simulink library "NxtrNvM"  (R2013b)
settings: Solver=ode45  StartTime=0.0  StopTime=10.0  RelTol=1e-3
settings Model: Creator=cz7lt6  LastModifiedBy=DZ1YRM

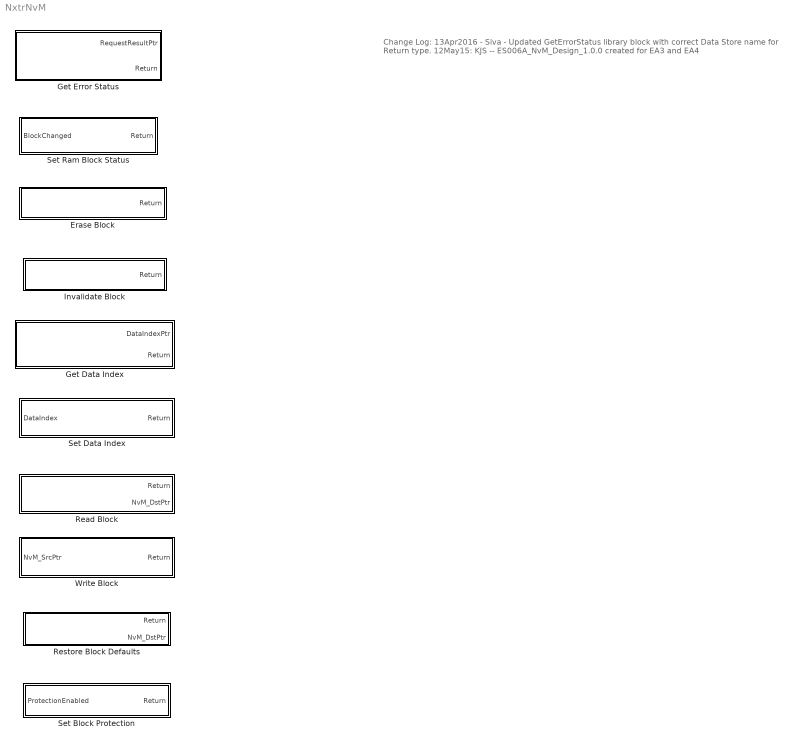
== system NxtrNvM ==
  note: Change Log:
      |
      |  13Apr2016 - Siva - Updated GetErrorStatus library block with correct Data Store name for Return type.
      |
      | 12May15: KJS -- ES006A_NvM_Design_1.0.0 created for EA3 and EA4
  Erase Block : Subsystem  mask(NvM EraseBlock){FuncName=Erase Block, NvMBlockName=, VoidFuncRtn=off, Return_DSN=NvMEraseBlk_Return}
      mask prompts: FuncName "%<FuncName>"; NvMBlockName "NvM Block Name"; VoidFuncRtn "Cast Function Return to Void"; Return_DSN "Data Store for Return"
      mask help: Click on Help for more details with respect to this function.
      mask init:
      | blk = [gcb '/Return'];
      | blkPos = get_param(blk, 'Position');
      | blkOri = get_param(blk, 'Orientation');
      | blkType = get_param(blk, 'BlockType');
      | 
      | if VoidFuncRtn
      |     if strcmp(blkType,'Outport')
      |         % Remove port and replace with terminator in the same location
      |         delete_block(blk);
      |         add_block('built-in/Terminator',blk,'Position',blkPos,...
      |                   'Orientation',blkOri);
      |         % Remove port and replace with terminator in the same location
      |         add_block('built-in/DataStoreMemory',[gcb '/Memory']);
      |         StoreName = get_param([gcb '/NvMEraseBlock_Return'],'DataStoreName');
      |         set_param([gcb '/Memory'],'DataStoreName',StoreName);
      |         
      |         % Add input port and terminate it
      |         add_block('built-in/Inport', [gcb '/CallFunction']);
      |         add_block('built-in/Terminator', [gcb '/CallFuncTerm']);
      |         add_line(gcb, 'CallFunction/1', 'CallFuncTerm/1',...
      |                  'autorouting', 'on');
      |         
      |         % Diable changes to Return data store
      |         set_param(gcb,'MaskEnableString','on,on,on,off');
      |     end
      | else
      |     if strcmp(blkType, 'Terminator')
      |         % Remove terminator and replace with outport
      |         delete_block(blk);
      |         add_block('built-in/Outport',blk,'Position',blkPos,...
      |                   'Orientation',blkOri);
      |         delete_block([gcb '/Memory']);
      |         
      |         %Remove input ports and connection
      |         delete_line(gcb, 'CallFunction/1', 'CallFuncTerm/1');
      |         delete_block([gcb '/CallFunction']);
      |         delete_block([gcb '/CallFuncTerm']);
      |         
      |         % Enable all fields in mask
      |         set_param(gcb,'MaskEnableString','on,on,on,on');
      |     end
      | end
      | %END%
      settings: AttributesFormatString=%<FuncName>
      mask Help: eval('web(NvMLibHelp(''EraseBlock.html''))')
      mask TypeOptions Return_DSN: NvMEraseBlock_Return/DataStoreName
      mask Display:
      | % Adjust ports based on mask configuration.
      | if VoidFuncRtn
      |     % No 'Return' port
      |     port_label('input',1,'CallFunction');
      | else
      |     port_label('output',1,'Return');
      | end
      | 
      | % Check NvM Block Name parameter
      | if isempty(NvMBlockName)
      |     NvMBlockName = 'Undefined NvM Block';
      |     color('red');
      | end
      | text(0.02,0.95,[NvMBlockName],...
      |      'horizontalAlignment', 'left',...
      |      'verticalAlignment','top');
  Get Data Index : Subsystem  mask(NvM GetDataIndex){FuncName=Get Data Index, NvMBlockName=, VoidFuncRtn=off, DataIndexPtr_DSN=DataIndexPtr, Return_DSN=NvMGDI_Return}
      mask prompts: FuncName "%<FuncName>"; NvMBlockName "NvM Block Name"; VoidFuncRtn "Cast Function Return to Void"; DataIndexPtr_DSN "Data Store for DataIndexPtr"; Return_DSN "Data Store for Return"
      mask help: Click on Help for more details with respect to this function.
      mask init:
      | blk = [gcb '/Return'];
      | blkPos = get_param(blk, 'Position');
      | blkOri = get_param(blk, 'Orientation');
      | blkType = get_param(blk, 'BlockType');
      | 
      | if VoidFuncRtn
      |     if strcmp(blkType,'Outport')
      |         % Remove port and replace with terminator in the same location
      |         delete_block(blk);
      |         add_block('built-in/Terminator',blk,'Position',blkPos,...
      |                   'Orientation',blkOri);
      |         
      |         % Add internal data store to prevent simulation errors
      |         add_block('built-in/DataStoreMemory',[gcb '/Memory']);
      |         
      |         % Give it the same name as the configured value
      |         StoreName = get_param([gcb '/NvMGDI_Return'],'DataStoreName');
      |         set_param([gcb '/Memory'],'DataStoreName',StoreName);
      | 
      |         % Turn off field in mask to prevent changes.
      |         set_param(gcb,'MaskEnableString','on,on,on,on,off')
      |     end
      | else
      |     if strcmp(blkType, 'Terminator')
      |         % Remove terminator and replace with outport
      |         delete_block(blk);
      |         add_block('built-in/Outport',blk,'Position',blkPos,...
      |                   'Orientation',blkOri);
      |         
      |         % Remove internal data store
      |         delete_block([gcb '/Memory']);
      |         
      |         % Enable field in mask to allow changes 
      |         set_param(gcb,'MaskEnableString','on,on,on,on,on')
      |     end
      | end
      settings: AttributesFormatString=%<FuncName>
      mask Help: eval('web(NvMLibHelp(''GetDataIndex.html''))')
      mask TypeOptions DataIndexPtr_DSN: NvMGDI_DataIndexPtr/DataStoreName
      mask TypeOptions Return_DSN: NvMGDI_Return/DataStoreName
      mask Display:
      | % Adjust ports based on mask configuration.
      | if VoidFuncRtn
      |     port_label('output',1,'DataIndexPtr');
      | else
      |     port_label('output',1,'DataIndexPtr');
      |     port_label('output',2,'Return');
      | end
      | 
      | % Check NvM Block Name parameter
      | if isempty(NvMBlockName)
      |     NvMBlockName = 'Undefined NvM Block';
      |     color('red');
      | end
      | text(0.02,0.95,[NvMBlockName],...
      |      'horizontalAlignment', 'left',...
      |      'verticalAlignment','top');
  Get Error Status : Subsystem  TreatAsAtomicUnit=on  mask(NvM GetErrorStatus){FuncName=Get Error Status, NvMBlockName=, VoidFuncRtn=off, ReqResPtr_DSN=NvMGES_ReqResPtr, Return_DSN=NvMGES_Return}
      mask prompts: FuncName "%<FuncName>"; NvMBlockName "NvM Block Name"; VoidFuncRtn "Cast Function Return to Void"; ReqResPtr_DSN "Data Store for ReqResPtr"; Return_DSN "Data Store for Return"
      mask help: Click on Help for more details with respect to this function.
      mask init:
      | blk = [gcb '/Return'];
      | blkPos = get_param(blk, 'Position');
      | blkOri = get_param(blk, 'Orientation');
      | blkType = get_param(blk, 'BlockType');
      | 
      | if VoidFuncRtn
      |     if strcmp(blkType,'Outport')
      |         % Remove port and replace with terminator in the same location
      |         delete_block(blk);
      |         add_block('built-in/Terminator',blk,'Position',blkPos,...
      |                   'Orientation',blkOri);
      |         % Add internal data store to prevent simulation errors
      |         add_block('built-in/DataStoreMemory',[gcb '/Memory']);
      |         
      |         % Give it the same name as the configured value
      |         StoreName = get_param([gcb '/NvMGES_Return'],'DataStoreName');
      |         set_param([gcb '/Memory'],'DataStoreName',StoreName);
      |         
      |         % Turn off field in mask to prevent changes.
      |         set_param(gcb,'MaskEnableString','on,on,on,on,off')
      |     end
      | else
      |     if strcmp(blkType, 'Terminator')
      |         % Remove terminator and replace with outport
      |         delete_block(blk);
      |         add_block('built-in/Outport',blk,'Position',blkPos,...
      |                   'Orientation',blkOri);
      |         
      |         % Remove internal data store
      |         delete_block([gcb '/Memory']);
      |         
      |         % Enable field in mask to allow changes 
      |         set_param(gcb,'MaskEnableString','on,on,on,on,on')
      |     end
      | end
      | %END%
      settings: AttributesFormatString=%<FuncName>
      mask Help: eval('web(NvMLibHelp(''GetErrorStatus.html''))')
      mask TypeOptions ReqResPtr_DSN: NvMGES_ReqResPtr/DataStoreName
      mask TypeOptions Return_DSN: NvMGES_Return/DataStoreName
      mask Display:
      | % Adjust ports based on mask configuration.
      | if VoidFuncRtn
      |     % No 'Return' port
      |     port_label('output',1,'ReqResPtr');
      | else
      |     port_label('output',1,'ReqResPtr');
      |     port_label('output',2,'Return');
      | end
      | 
      | % Check NvM Block Name parameter
      | if isempty(NvMBlockName)
      |     NvMBlockName = 'Undefined NvM Block';
      |     color('red');
      | end
      | text(0.02,0.95,[NvMBlockName],...
      |      'horizontalAlignment', 'left',...
      |      'verticalAlignment','top');
  Invalidate Block : Subsystem  mask(NvM InvalidateBlock){FuncName=Invalidate Block, NvMBlockName=, VoidFuncRtn=off, Return_DSN=NvMInvalidateBlk_Return}
      mask prompts: FuncName "%<FuncName>"; NvMBlockName "NvM Block Name"; VoidFuncRtn "Cast Function Return to Void"; Return_DSN "Data Store for Return"
      mask help: Click on Help for more details with respect to this function.
      mask init:
      | blk = [gcb '/Return'];
      | blkPos = get_param(blk, 'Position');
      | blkOri = get_param(blk, 'Orientation');
      | blkType = get_param(blk, 'BlockType');
      | 
      | if VoidFuncRtn
      |     if strcmp(blkType,'Outport')
      |         % Remove port and replace with terminator in the same location
      |         delete_block(blk);
      |         add_block('built-in/Terminator',blk,'Position',blkPos,...
      |                   'Orientation',blkOri);
      |         % Remove port and replace with terminator in the same location
      |         add_block('built-in/DataStoreMemory',[gcb '/Memory']);
      |         StoreName = get_param([gcb '/NvMInvalidateBlock_Return'],'DataStoreName');
      |         set_param([gcb '/Memory'],'DataStoreName',StoreName);
      |         
      |         % Add input port and terminate it
      |         add_block('built-in/Inport', [gcb '/CallFunction']);
      |         add_block('built-in/Terminator', [gcb '/CallFuncTerm']);
      |         add_line(gcb, 'CallFunction/1', 'CallFuncTerm/1',...
      |                  'autorouting', 'on');
      |         
      |         % Diable changes to Return data store
      |         set_param(gcb,'MaskEnableString','on,on,on,off');
      |     end
      | else
      |     if strcmp(blkType, 'Terminator')
      |         % Remove terminator and replace with outport
      |         delete_block(blk);
      |         add_block('built-in/Outport',blk,'Position',blkPos,...
      |                   'Orientation',blkOri);
      |         delete_block([gcb '/Memory']);
      |         
      |         %Remove input ports and connection
      |         delete_line(gcb, 'CallFunction/1', 'CallFuncTerm/1');
      |         delete_block([gcb '/CallFunction']);
      |         delete_block([gcb '/CallFuncTerm']);
      |         
      |         % Enable all fields in mask
      |         set_param(gcb,'MaskEnableString','on,on,on,on');
      |     end
      | end
      | %END%
      settings: AttributesFormatString=%<FuncName>
      mask Help: eval('web(NvMLibHelp(''InvalidateBlock.html''))')
      mask TypeOptions Return_DSN: NvMInvalidateBlock_Return/DataStoreName
      mask Display:
      | % Adjust ports based on mask configuration.
      | if VoidFuncRtn
      |     % No 'Return' port
      |     port_label('input',1,'CallFunction');
      | else
      |     port_label('output',1,'Return');
      | end
      | 
      | % Check NvM Block Name parameter
      | if isempty(NvMBlockName)
      |     NvMBlockName = 'Undefined NvM Block';
      |     color('red');
      | end
      | text(0.02,0.95,[NvMBlockName],...
      |      'horizontalAlignment', 'left',...
      |      'verticalAlignment','top');
  Read Block : Subsystem  mask(NvM ReadBlock){FuncName=Read Block, NvMBlockName=, VoidFuncRtn=off, NvMDstPtr_DSN=NvM_DstPtr, Return_DSN=NvMReadBlock_Return, NullPtr=off}
      mask prompts: FuncName "%<FuncName>"; NvMBlockName "NvM Block Name"; VoidFuncRtn "Cast Function Return to Void"; NvMDstPtr_DSN "Data Store for NvM_DstPtr"; Return_DSN "Data Store for Return"; NullPtr "Set Output to NULL_PTR"
      mask help: Click on Help for more details with respect to this function.
      mask init:
      | blk = [gcb '/Return'];
      | blkPos = get_param(blk, 'Position');
      | blkOri = get_param(blk, 'Orientation');
      | blkType = get_param(blk, 'BlockType');
      | 
      | if VoidFuncRtn
      |     if strcmp(blkType,'Outport')
      |         % Remove port and replace with terminator in the same location
      |         delete_block(blk);
      |         add_block('built-in/Terminator',blk,'Position',blkPos,...
      |                   'Orientation',blkOri);
      |               
      |         % Add internal data store to prevent simulation errors
      |         add_block('built-in/DataStoreMemory',[gcb '/Memory']);
      |         
      |         % Give it the same name as the configured value
      |         StoreName = get_param([gcb '/NvMReadBlock_Return'],'DataStoreName');
      |         set_param([gcb '/Memory'],'DataStoreName',StoreName);
      |         
      |         % Turn off field in mask to prevent changes.
      |         set_param(gcb,'MaskEnableString','on,on,on,on,off,on')
      |     end
      | else
      |     if strcmp(blkType, 'Terminator')
      |         % Remove terminator and replace with outport
      |         delete_block(blk);
      |         add_block('built-in/Outport',blk,'Position',blkPos,...
      |                   'Orientation',blkOri);
      |         
      |         % Remove internal data store
      |         delete_block([gcb '/Memory']);
      |         
      |         % Enable field in mask to allow changes 
      |         set_param(gcb,'MaskEnableString','on,on,on,on,on,on')
      |     end
      | end
      | 
      | blk = [gcb '/NvM_DstPtr'];
      | blkPos = get_param(blk, 'Position');
      | blkOri = get_param(blk, 'Orientation');
      | blkType = get_param(blk, 'BlockType');
      | 
      | if NullPtr
      |     if strcmp(blkType,'Outport')
      |         % Remove port and replace with terminator in the same location
      |         delete_block(blk);
      |         add_block('built-in/Terminator',blk,'Position',blkPos,...
      |                   'Orientation',blkOri);
      |               
      |         % Add internal data store to prevent simulation errors
      |         add_block('built-in/DataStoreMemory',[gcb '/Memory2']);
      |         
      |         % Give it the same name as the configured value
      |         StoreName = get_param([gcb '/NvMReadBlock_DstPtr'],'DataStoreName');
      |         set_param([gcb '/Memory2'],'DataStoreName',StoreName);
      |         
      |         % Add input port and connect it to a terminator
      |         add_block('built-in/Inport',[gcb '/CallFunction']);
      |         add_block('built-in/Terminator', [gcb '/CallFuncTerm']);
      |         add_line(gcb, 'CallFunction/1', 'CallFuncTerm/1',...
      |                  'autorouting','on');
      |     end
      | else
      |     if strcmp(blkType, 'Terminator')
      |         % Remove terminator and replace with outport
      |         delete_block(blk);
      |         add_block('built-in/Outport',blk,'Position',blkPos,...
      |                   'Orientation',blkOri);
      |         
      |         % Remove internal data store
      |         delete_block([gcb '/Memory2']);
      |         
      |         % Remove connection and then remove ports
      |         delete_line(gcb, 'CallFunction/1', 'CallFuncTerm/1');
      |         delete_block([gcb '/CallFunction']);
      |         delete_block([gcb '/CallFuncTerm']);
      |     end
      | end
      settings: AttributesFormatString=%<FuncName>
      mask Help: eval('web(NvMLibHelp(''ReadBlock.html''))')
      mask TypeOptions NvMDstPtr_DSN: NvMReadBlock_DstPtr/DataStoreName
      mask TypeOptions Return_DSN: NvMReadBlock_Return/DataStoreName
      mask DialogControl Control2 Prompt: If the following box is checked, NULL_PTR is passed to the ReadBlock function. NULL_PTR will cause the NvM to write to the configured RAM address for the NvM block, which is typically the PIM defined in the M-file. With this enabled, the input to this block shall be interpreted as when the function shall be called, hence the port name changes to CallFunction and becomes an input.
      mask Display:
      | % Adjust ports based on mask configuration.
      | if NullPtr
      |     port_label('input',1,'CallFunction');
      | else
      |     port_label('output',1,'NvM_DstPtr');
      | end
      | 
      | if VoidFuncRtn
      | else
      |     if NullPtr
      |         port_label('output',1,'Return');
      |     else
      |         port_label('output',2,'Return');
      |     end
      | end
      | 
      | % Check NvM Block Name parameter
      | if isempty(NvMBlockName)
      |     NvMBlockName = 'Undefined NvM Block';
      |     color('red');
      | end
      | text(0.02,0.95,[NvMBlockName],...
      |      'horizontalAlignment', 'left',...
      |      'verticalAlignment','top');
  Restore Block Defaults : Subsystem  mask(NvM RestoreBlockDefaults){FuncName=Restore Block Defaults, NvMBlockName=, VoidFuncRtn=off, NvMDstPtr_DSN=NvMRBD_DstPtr, Return_DSN=NvMRBD_Return, NullPtr=off}
      mask prompts: FuncName "%<FuncName>"; NvMBlockName "NvM Block Name"; VoidFuncRtn "Cast Function Return to Void"; NvMDstPtr_DSN "Data Store for NvM_DstPtr"; Return_DSN "Data Store for Return"; NullPtr "Set Output to NULL_PTR"
      mask help: Click on Help for more details with respect to this function.
      mask init:
      | blk = [gcb '/Return'];
      | blkPos = get_param(blk, 'Position');
      | blkOri = get_param(blk, 'Orientation');
      | blkType = get_param(blk, 'BlockType');
      | 
      | if VoidFuncRtn
      |     if strcmp(blkType,'Outport')
      |         % Remove port and replace with terminator in the same location
      |         delete_block(blk);
      |         add_block('built-in/Terminator',blk,'Position',blkPos,...
      |                   'Orientation',blkOri);
      |               
      |         % Add internal data store to prevent simulation errors
      |         add_block('built-in/DataStoreMemory',[gcb '/Memory']);
      |         
      |         % Give it the same name as the configured value
      |         StoreName = get_param([gcb '/NvMRBD_Return'],'DataStoreName');
      |         set_param([gcb '/Memory'],'DataStoreName',StoreName);
      |         
      |         % Turn off field in mask to prevent changes.
      |         set_param(gcb,'MaskEnableString','on,on,on,on,off,on')
      |     end
      | else
      |     if strcmp(blkType, 'Terminator')
      |         % Remove terminator and replace with outport
      |         delete_block(blk);
      |         add_block('built-in/Outport',blk,'Position',blkPos,...
      |                   'Orientation',blkOri);
      |         
      |         % Remove internal data store
      |         delete_block([gcb '/Memory']);
      |         
      |         % Enable field in mask to allow changes 
      |         set_param(gcb,'MaskEnableString','on,on,on,on,on,on')
      |     end
      | end
      | 
      | blk = [gcb '/NvM_DstPtr'];
      | blkPos = get_param(blk, 'Position');
      | blkOri = get_param(blk, 'Orientation');
      | blkType = get_param(blk, 'BlockType');
      | 
      | if NullPtr
      |     if strcmp(blkType,'Outport')
      |         % Remove port and replace with terminator in the same location
      |         delete_block(blk);
      |         add_block('built-in/Terminator',blk,'Position',blkPos,...
      |                   'Orientation',blkOri);
      |               
      |         % Add internal data store to prevent simulation errors
      |         add_block('built-in/DataStoreMemory',[gcb '/Memory2']);
      |         
      |         % Give it the same name as the configured value
      |         StoreName = get_param([gcb '/NvMRBD_DstPtr'],'DataStoreName');
      |         set_param([gcb '/Memory2'],'DataStoreName',StoreName);
      |         
      |         % Add input port and connect it to a terminator
      |         add_block('built-in/Inport',[gcb '/CallFunction']);
      |         add_block('built-in/Terminator', [gcb '/CallFuncTerm']);
      |         add_line(gcb, 'CallFunction/1', 'CallFuncTerm/1',...
      |                  'autorouting','on');
      |     end
      | else
      |     if strcmp(blkType, 'Terminator')
      |         % Remove terminator and replace with outport
      |         delete_block(blk);
      |         add_block('built-in/Outport',blk,'Position',blkPos,...
      |                   'Orientation',blkOri);
      |         
      |         % Remove internal data store
      |         delete_block([gcb '/Memory2']);
      |         
      |         % Remove connection and then remove ports
      |         delete_line(gcb, 'CallFunction/1', 'CallFuncTerm/1');
      |         delete_block([gcb '/CallFunction']);
      |         delete_block([gcb '/CallFuncTerm']);
      |     end
      | end
      settings: AttributesFormatString=%<FuncName>
      mask Help: eval('web(NvMLibHelp(''RestoreBlockDefaults.html''))')
      mask TypeOptions NvMDstPtr_DSN: NvMRBD_DstPtr/DataStoreName
      mask TypeOptions Return_DSN: NvMRBD_Return/DataStoreName
      mask DialogControl Control2 Prompt: If the following box is checked, NULL_PTR is passed to the ReadBlock function. NULL_PTR will cause the NvM to write to the configured RAM address for the NvM block, which is typically the PIM defined in the M-file. With this enabled, the input to this block shall be interpreted as when the function shall be called, hence the port name changes to CallFunction and becomes an input.
      mask Display:
      | % Adjust ports based on mask configuration.
      | if NullPtr
      |     port_label('input',1,'CallFunction');
      | else
      |     port_label('output',1,'NvM_DstPtr');
      | end
      | 
      | if VoidFuncRtn
      | else
      |     if NullPtr
      |         port_label('output',1,'Return');
      |     else
      |         port_label('output',2,'Return');
      |     end
      | end
      | 
      | % Check NvM Block Name parameter
      | if isempty(NvMBlockName)
      |     NvMBlockName = 'Undefined NvM Block';
      |     color('red');
      | end
      | text(0.02,0.95,[NvMBlockName],...
      |      'horizontalAlignment', 'left',...
      |      'verticalAlignment','top');
  Set Block Protection : Subsystem  mask(NvM SetBlockProtection){FuncName=Set Block Protection, NvMBlockName=, VoidFuncRtn=off, ProtectionEnabled_DSN=ProtectionEnabled, Return_DSN=NvMSBP_Return}
      mask prompts: FuncName "%<FuncName>"; NvMBlockName "NvM Block Name"; VoidFuncRtn "Cast Function Return to Void"; ProtectionEnabled_DSN "Data Store for Protection Enabled"; Return_DSN "Data Store for Return"
      mask help: Click on Help for more details with respect to this function.
      mask init:
      | blk = [gcb '/Return'];
      | blkPos = get_param(blk, 'Position');
      | blkOri = get_param(blk, 'Orientation');
      | blkType = get_param(blk, 'BlockType');
      | 
      | if VoidFuncRtn
      |     if strcmp(blkType,'Outport')
      | % Remove port and replace with terminator in the same location
      |         delete_block(blk);
      |         add_block('built-in/Terminator',blk,'Position',blkPos,...
      |                   'Orientation',blkOri);
      |         
      |         % Add internal data store to prevent simulation errors
      |         add_block('built-in/DataStoreMemory',[gcb '/Memory']);
      |         
      |         % Give it the same name as the configured value
      |         StoreName = get_param([gcb '/NvMSBP_Return'],'DataStoreName');
      |         set_param([gcb '/Memory'],'DataStoreName',StoreName);
      | 
      |         % Turn off field in mask to prevent changes.
      |         set_param(gcb,'MaskEnableString','on,on,on,on,off');
      |     end
      | else
      |    if strcmp(blkType, 'Terminator')
      |         % Remove terminator and replace with outport
      |         delete_block(blk);
      |         add_block('built-in/Outport',blk,'Position',blkPos,...
      |                   'Orientation',blkOri);
      |         
      |         % Remove internal data store
      |         delete_block([gcb '/Memory']);
      |         
      |         % Enable field in mask to allow changes 
      |         set_param(gcb,'MaskEnableString','on,on,on,on,on');
      |    end
      | end
      settings: AttributesFormatString=%<FuncName>
      mask Help: eval('web(NvMLibHelp(''SetBlockProtection.html''))')
      mask TypeOptions ProtectionEnabled_DSN: NvMSBP_ProtectionEnabled/DataStoreName
      mask TypeOptions Return_DSN: NvMSBP_Return/DataStoreName
      mask Display:
      | % Adjust ports based on mask configuration.
      | if VoidFuncRtn
      |     % No 'Return' port
      |     port_label('input',1,'ProtectionEnabled');
      | else
      |     port_label('output',1,'Return');
      |     port_label('input',1,'ProtectionEnabled');
      | end
      | 
      | % Check Block Name parameter
      | if isempty(NvMBlockName)
      |     NvMBlockName = 'Undefined NvM Block';
      |     color('red');
      | end
      | text(0.02,0.95,[NvMBlockName],...
      |      'horizontalAlignment', 'left',...
      |      'verticalAlignment','top');
  Set Data Index : Subsystem  mask(NvM SetDataIndex){FuncName=Set Data Index, NvMBlockName=, VoidFuncRtn=off, DataIndex_DSN=DataIndex, Return_DSN=NvMSDI_Return}
      mask prompts: FuncName "%<FuncName>"; NvMBlockName "NvM Block Name"; VoidFuncRtn "Cast Function Return to Void"; DataIndex_DSN "Data Store for Data Index"; Return_DSN "Data Store for Return"
      mask help: Click on Help for more details with respect to this function.
      mask init:
      | blk = [gcb '/Return'];
      | blkPos = get_param(blk, 'Position');
      | blkOri = get_param(blk, 'Orientation');
      | blkType = get_param(blk, 'BlockType');
      | 
      | if VoidFuncRtn
      |     if strcmp(blkType,'Outport')
      |         % Remove port and replace with terminator in the same location
      |         delete_block(blk);
      |         add_block('built-in/Terminator',blk,'Position',blkPos,...
      |                   'Orientation',blkOri);
      |         
      |         % Add internal data store to prevent simulation errors
      |         add_block('built-in/DataStoreMemory',[gcb '/Memory']);
      |         
      |         % Give it the same name as the configured value
      |         StoreName = get_param([gcb '/NvMSDI_Return'],'DataStoreName');
      |         set_param([gcb '/Memory'],'DataStoreName',StoreName);
      | 
      |         % Turn off field in mask to prevent changes.
      |         set_param(gcb,'MaskEnableString','on,on,on,on,off');
      |     end
      | else
      |    if strcmp(blkType, 'Terminator')
      |         % Remove terminator and replace with outport
      |         delete_block(blk);
      |         add_block('built-in/Outport',blk,'Position',blkPos,...
      |                   'Orientation',blkOri);
      |         
      |         % Remove internal data store
      |         delete_block([gcb '/Memory']);
      |         
      |         % Enable field in mask to allow changes 
      |         set_param(gcb,'MaskEnableString','on,on,on,on,on');
      |    end
      | end
      settings: AttributesFormatString=%<FuncName>
      mask Help: eval('web(NvMLibHelp(''SetDataIndex.html''))')
      mask TypeOptions DataIndex_DSN: NvMSDI_DataIndex/DataStoreName
      mask TypeOptions Return_DSN: NvMSDI_Return/DataStoreName
      mask Display:
      | % Adjust ports based on mask configuration.
      | if VoidFuncRtn
      |     % No 'Return' port
      |     port_label('input',1,'DataIndex');
      | else
      |     port_label('output',1,'Return');
      |     port_label('input',1,'DataIndex');
      | end
      | 
      | % Check Block Name parameter
      | if isempty(NvMBlockName)
      |     NvMBlockName = 'Undefined NvM Block';
      |     color('red');
      | end
      | text(0.02,0.95,[NvMBlockName],...
      |      'horizontalAlignment', 'left',...
      |      'verticalAlignment','top');
  Set Ram Block Status : Subsystem  mask(NvM SetRamBlockStatus){FuncName=Set Ram Block Status, NvMBlockName=, VoidFuncRtn=off, BlockChanged_DSN=NvMSRBS_BlockChanged, Return_DSN=NvMSRBS_Return}
      mask prompts: FuncName "%<FuncName>"; NvMBlockName "NvM Block Name"; VoidFuncRtn "Cast Function Return to Void"; BlockChanged_DSN "Data Store for Block Changed"; Return_DSN "Data Store for Return"
      mask help: Click on Help for more details with respect to this function.
      mask init:
      | blk = [gcb '/Return'];
      | blkPos = get_param(blk, 'Position');
      | blkOri = get_param(blk, 'Orientation');
      | blkType = get_param(blk, 'BlockType');
      | 
      | if VoidFuncRtn
      |     if strcmp(blkType,'Outport')
      |         % Remove port and replace with terminator in the same location
      |         delete_block(blk);
      |         add_block('built-in/Terminator',blk,'Position',blkPos,...
      |                   'Orientation',blkOri);
      |         % Add internal data store to prevent simulation errors
      |         add_block('built-in/DataStoreMemory',[gcb '/Memory']);
      |         StoreName = get_param([gcb '/NvMSRBS_Return'],'DataStoreName');
      |         set_param([gcb '/Memory'],'DataStoreName',StoreName);
      |         
      |         % Diable changes to Return data store
      |         set_param(gcb,'MaskEnableString','on,on,on,on,off');
      |     end
      | else
      |    if strcmp(blkType, 'Terminator')
      |        % Remove terminator and replace with outport
      |        delete_block(blk);
      |        add_block('built-in/Outport',blk,'Position',blkPos,...
      |                   'Orientation',blkOri);
      |        
      |        % Remove internal data store
      |        delete_block([gcb '/Memory']);
      |        
      |        % Enable all fields in mask
      |        set_param(gcb,'MaskEnableString','on,on,on,on,on');
      |    end
      | end
      | %END%
      settings: AttributesFormatString=%<FuncName>
      mask Help: eval('web(NvMLibHelp(''SetRamBlockStatus.html''))')
      mask TypeOptions BlockChanged_DSN: NvMSRBS_BlockChanged/DataStoreName
      mask TypeOptions Return_DSN: NvMSRBS_Return/DataStoreName
      mask Display:
      | % Adjust ports based on mask configuration.
      | if VoidFuncRtn
      |     % No 'Return' port
      |     port_label('input',1,'BlockChanged');
      | else
      |     port_label('input',1,'BlockChanged');
      |     port_label('output',1,'Return');
      | end
      | 
      | % Check NvM Block Name parameter
      | if isempty(NvMBlockName)
      |     NvMBlockName = 'Undefined NvM Block';
      |     color('red');
      | end
      | text(0.02,0.95,[NvMBlockName],...
      |      'horizontalAlignment', 'left',...
      |      'verticalAlignment','top');
  Write Block : Subsystem  mask(NvM WriteBlock){FuncName=Write Block, NvMBlockName=, VoidFuncRtn=off, SrcPtr_DSN=NvM_SrcPtr, Return_DSN=NvMWriteBlock_Return, NullPtr=off}
      mask prompts: FuncName "%<FuncName>"; NvMBlockName "NvM Block Name"; VoidFuncRtn "Cast Function Return to Void"; SrcPtr_DSN "Data Store for SrcPtr"; Return_DSN "Data Store for Return"; NullPtr "Set Input to NULL_PTR"
      mask help: Click on Help for more details with respect to this function.
      mask init:
      | blk = [gcb '/Return'];
      | blkPos = get_param(blk, 'Position');
      | blkOri = get_param(blk, 'Orientation');
      | blkType = get_param(blk, 'BlockType');
      | 
      | if VoidFuncRtn
      |     if strcmp(blkType,'Outport')
      |         % Remove port and replace with terminator in the same location
      |         delete_block(blk);
      |         add_block('built-in/Terminator',blk,'Position',blkPos,...
      |                   'Orientation',blkOri);
      |               
      |         % Add internal data store to prevent simulation errors
      |         add_block('built-in/DataStoreMemory',[gcb '/Memory']);
      |         
      |         % Give it the same name as the configured value
      |         StoreName = get_param([gcb '/NvMWriteBlock_Return'],'DataStoreName');
      |         set_param([gcb '/Memory'],'DataStoreName',StoreName);
      |         
      |         % Turn off field in mask to prevent changes.
      |         if NullPtr
      |             set_param(gcb,'MaskEnableString','on,on,on,off,off,on');
      |         else
      |             set_param(gcb,'MaskEnableString','on,on,on,on,off,on');
      |         end
      |     end
      | else
      |    if strcmp(blkType, 'Terminator')
      |         % Remove terminator and replace with outport
      |         delete_block(blk);
      |         add_block('built-in/Outport',blk,'Position',blkPos,...
      |                   'Orientation',blkOri);
      |         
      |         % Remove internal data store
      |         delete_block([gcb '/Memory']);
      |         
      |         % Enable field in mask to allow changes 
      |         if NullPtr
      |             set_param(gcb,'MaskEnableString','on,on,on,off,on,on');
      |         else
      |             set_param(gcb,'MaskEnableString','on,on,on,on,on,on');
      |         end
      |    end
      | end
      | 
      | %Same process for NullPtr on the input side. 
      | blk = [gcb '/NvMWriteBlock_SrcPtr'];
      | blkPos = get_param(blk, 'Position');
      | blkOri = get_param(blk, 'Orientation');
      | blkType = get_param(blk, 'BlockType');
      | 
      | if NullPtr
      |     if strcmp(blkType,'DataStoreWrite')
      |         % Remove port and replace with terminator
      |         delete_block(blk);
      |         add_block('built-in/Terminator',blk,'Position',blkPos,...
      |                   'Orientation',blkOri);
      |         if VoidFuncRtn
      |             set_param(gcb,'MaskEnableString','on,on,on,off,off,on');
      |         else
      |             set_param(gcb,'MaskEnableString','on,on,on,off,on,on');
      |         end
      |     end
      | else
      |    if strcmp(blkType, 'Terminator')
      |        % Remove terminator and replace with outport
      |        delete_block(blk);
      |        add_block('built-in/DataStoreWrite',blk,'Position',blkPos,...
      |                   'Orientation',blkOri);
      |        set_param(blk,'DataStoreName',SrcPtr_DSN);
      |         if VoidFuncRtn
      |             set_param(gcb,'MaskEnableString','on,on,on,on,off,on');
      |         else
      |             set_param(gcb,'MaskEnableString','on,on,on,on,on,on');
      |         end
      |    end
      | end
      settings: AttributesFormatString=%<FuncName>
      mask Help: eval('web(NvMLibHelp(''WriteBlock.html''))')
      mask TypeOptions SrcPtr_DSN: NvMWriteBlock_SrcPtr/DataStoreName
      mask TypeOptions Return_DSN: NvMWriteBlock_Return/DataStoreName
      mask DialogControl Control2 Prompt: If the following box is checked, NULL_PTR is passed to the WriteBlock function. NULL_PTR will cause the NvM to read from the configured RAM address for the NvM block, which is typically the PIM defined in the M-file. With this enabled, the input to this block shall be interpreted as when the function shall be called, hence the port name changes to CallFunction.
      mask Display:
      | % Adjust ports based on mask configuration.
      | if VoidFuncRtn
      |     % No 'Return' port
      | else
      |     port_label('output',1,'Return');
      | end
      | 
      | if NullPtr
      |     port_label('input',1,'CallFunction');
      | else
      |     port_label('input',1,'NvM_SrcPtr');
      | end
      | 
      | % Check NvM Block Name parameter
      | if isempty(NvMBlockName)
      |     NvMBlockName = 'Undefined NvM Block';
      |     color('red');
      | end
      | text(0.02,0.95,[NvMBlockName],...
      |      'horizontalAlignment', 'left',...
      |      'verticalAlignment','top');

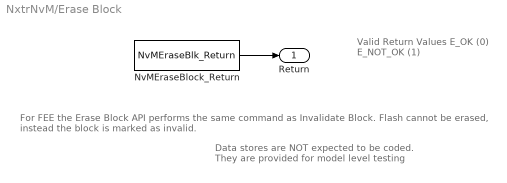
== system NxtrNvM/Erase Block ==
  note: For FEE the Erase Block API performs the same command as Invalidate Block. Flash cannot be erased, instead the block is marked as invalid.
  note: Valid Return Values
      | E_OK (0)
      | E_NOT_OK (1)
  note: Data stores are NOT expected to be coded.
      | They are provided for model level testing
  NvMEraseBlock_Return : DataStoreRead  DataStoreName=NvMEraseBlk_Return
  Return : Outport
  wires:
  NvMEraseBlock_Return/1 -> Return/1

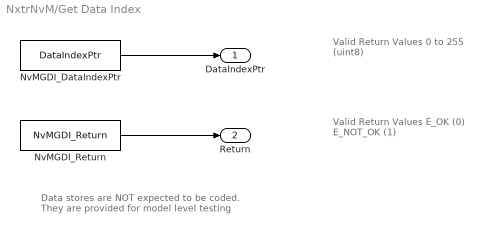
== system NxtrNvM/Get Data Index ==
  note: Valid Return Values
      | E_OK (0)
      | E_NOT_OK (1)
  note: Data stores are NOT expected to be coded.
      | They are provided for model level testing
  note: Valid Return Values
      | 0 to 255 (uint8)
  NvMGDI_DataIndexPtr : DataStoreRead  DataStoreName=DataIndexPtr
  NvMGDI_Return : DataStoreRead  DataStoreName=NvMGDI_Return
  DataIndexPtr : Outport
  Return : Outport  Port=2
  wires:
  NvMGDI_Return/1 -> Return/1
  NvMGDI_DataIndexPtr/1 -> DataIndexPtr/1

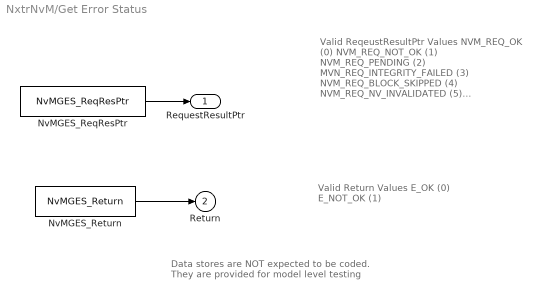
== system NxtrNvM/Get Error Status ==
  note: Valid Return Values
      | E_OK (0)
      | E_NOT_OK (1)
  note: Valid ReqeustResultPtr Values
      | NVM_REQ_OK (0)
      | NVM_REQ_NOT_OK (1)
      | NVM_REQ_PENDING (2)
      | MVN_REQ_INTEGRITY_FAILED (3)
      | NVM_REQ_BLOCK_SKIPPED (4)
      | NVM_REQ_NV_INVALIDATED (5)
      | NVM_REQ_CANCELLED (6)
      | NVM_REQ_REDUNDANCY_FAILED (7)
      | NVM_REQ_RESTORED_FROM_ROM (8)
  note: Data stores are NOT expected to be coded.
      | They are provided for model level testing
  NvMGES_ReqResPtr : DataStoreRead  DataStoreName=NvMGES_ReqResPtr
  NvMGES_Return : DataStoreRead  DataStoreName=NvMGES_Return
  RequestResultPtr : Outport
  Return : Outport  Port=2
  wires:
  NvMGES_Return/1 -> Return/1
  NvMGES_ReqResPtr/1 -> RequestResultPtr/1

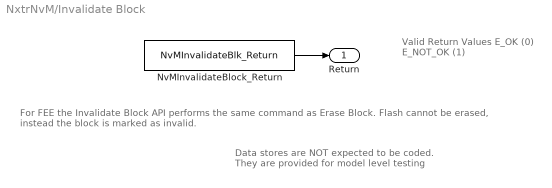
== system NxtrNvM/Invalidate Block ==
  note: Valid Return Values
      | E_OK (0)
      | E_NOT_OK (1)
  note: Data stores are NOT expected to be coded.
      | They are provided for model level testing
  note: For FEE the Invalidate Block API performs the same command as Erase Block. Flash cannot be erased, instead the block is marked as invalid.
  NvMInvalidateBlock_Return : DataStoreRead  DataStoreName=NvMInvalidateBlk_Return
  Return : Outport
  wires:
  NvMInvalidateBlock_Return/1 -> Return/1

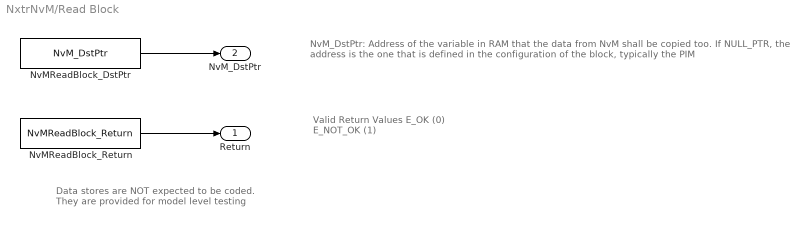
== system NxtrNvM/Read Block ==
  note: Valid Return Values
      | E_OK (0)
      | E_NOT_OK (1)
  note: NvM_DstPtr: Address of the variable in RAM that the data from NvM shall be copied too. If NULL_PTR, the address is the
      | one that is defined in the configuration of the block, typically the PIM
  note: Data stores are NOT expected to be coded.
      | They are provided for model level testing
  NvMReadBlock_DstPtr : DataStoreRead  DataStoreName=NvM_DstPtr
  NvMReadBlock_Return : DataStoreRead  DataStoreName=NvMReadBlock_Return
  Return : Outport
  NvM_DstPtr : Outport  Port=2
  wires:
  NvMReadBlock_Return/1 -> Return/1
  NvMReadBlock_DstPtr/1 -> NvM_DstPtr/1

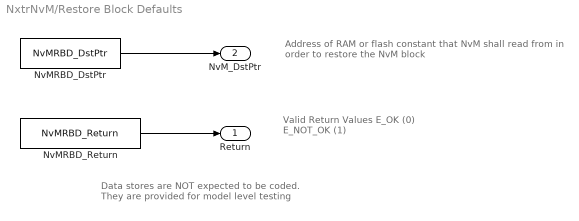
== system NxtrNvM/Restore Block Defaults ==
  note: Valid Return Values
      | E_OK (0)
      | E_NOT_OK (1)
  note: Address of RAM or flash constant that NvM shall read from
      | in order to restore the NvM block
  note: Data stores are NOT expected to be coded.
      | They are provided for model level testing
  NvMRBD_DstPtr : DataStoreRead  DataStoreName=NvMRBD_DstPtr
  NvMRBD_Return : DataStoreRead  DataStoreName=NvMRBD_Return
  Return : Outport
  NvM_DstPtr : Outport  Port=2
  wires:
  NvMRBD_Return/1 -> Return/1
  NvMRBD_DstPtr/1 -> NvM_DstPtr/1

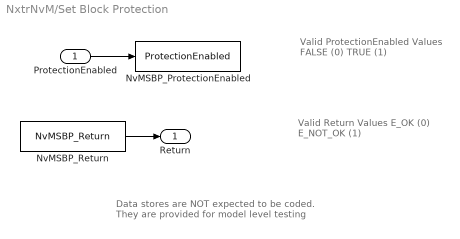
== system NxtrNvM/Set Block Protection ==
  note: Valid Return Values
      | E_OK (0)
      | E_NOT_OK (1)
  note: Valid ProtectionEnabled Values
      | FALSE (0)
      | TRUE (1)
  note: Data stores are NOT expected to be coded.
      | They are provided for model level testing
  ProtectionEnabled : Inport
  NvMSBP_ProtectionEnabled : DataStoreWrite  DataStoreName=ProtectionEnabled
  NvMSBP_Return : DataStoreRead  DataStoreName=NvMSBP_Return
  Return : Outport
  wires:
  ProtectionEnabled/1 -> NvMSBP_ProtectionEnabled/1
  NvMSBP_Return/1 -> Return/1

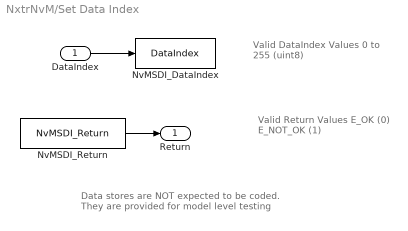
== system NxtrNvM/Set Data Index ==
  note: Valid Return Values
      | E_OK (0)
      | E_NOT_OK (1)
  note: Valid DataIndex Values
      | 0 to 255 (uint8)
  note: Data stores are NOT expected to be coded.
      | They are provided for model level testing
  DataIndex : Inport
  NvMSDI_DataIndex : DataStoreWrite  DataStoreName=DataIndex
  NvMSDI_Return : DataStoreRead  DataStoreName=NvMSDI_Return
  Return : Outport
  wires:
  DataIndex/1 -> NvMSDI_DataIndex/1
  NvMSDI_Return/1 -> Return/1

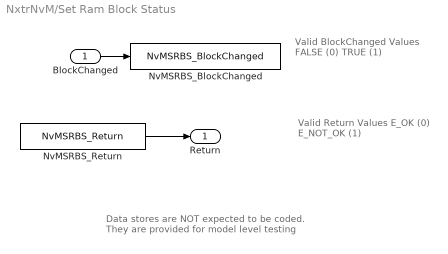
== system NxtrNvM/Set Ram Block Status ==
  note: Valid Return Values
      | E_OK (0)
      | E_NOT_OK (1)
  note: Valid BlockChanged Values
      | FALSE (0)
      | TRUE (1)
  note: Data stores are NOT expected to be coded.
      | They are provided for model level testing
  BlockChanged : Inport
  NvMSRBS_BlockChanged : DataStoreWrite  DataStoreName=NvMSRBS_BlockChanged
  NvMSRBS_Return : DataStoreRead  DataStoreName=NvMSRBS_Return
  Return : Outport
  wires:
  BlockChanged/1 -> NvMSRBS_BlockChanged/1
  NvMSRBS_Return/1 -> Return/1

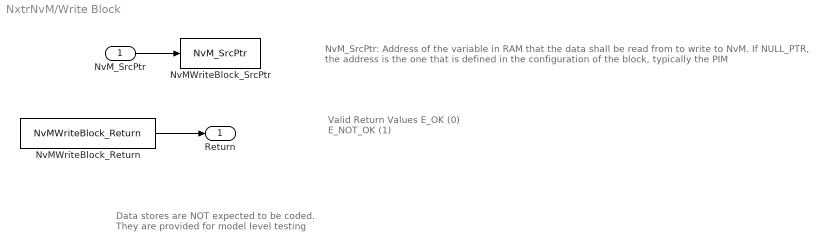
== system NxtrNvM/Write Block ==
  note: Valid Return Values
      | E_OK (0)
      | E_NOT_OK (1)
  note: NvM_SrcPtr: Address of the variable in RAM that the data shall be read from to write to NvM. If NULL_PTR, the address is the
      | one that is defined in the configuration of the block, typically the PIM
  note: Data stores are NOT expected to be coded.
      | They are provided for model level testing
  NvM_SrcPtr : Inport
  NvMWriteBlock_Return : DataStoreRead  DataStoreName=NvMWriteBlock_Return
  NvMWriteBlock_SrcPtr : DataStoreWrite  DataStoreName=NvM_SrcPtr
  Return : Outport
  wires:
  NvM_SrcPtr/1 -> NvMWriteBlock_SrcPtr/1
  NvMWriteBlock_Return/1 -> Return/1
